simulink model "Comparacao_tomada_de_corrente_mq"  (R2024a)
settings: Solver=FixedStepAuto  StartTime=0.0  StopTime=1  FixedStep=T  RelTol=1e-3
undefined symbols (not defined in the file): J, Kf, La, T, Te, Tm, Vn
settings Model: Creator=lpds  LastModifiedBy=lpds

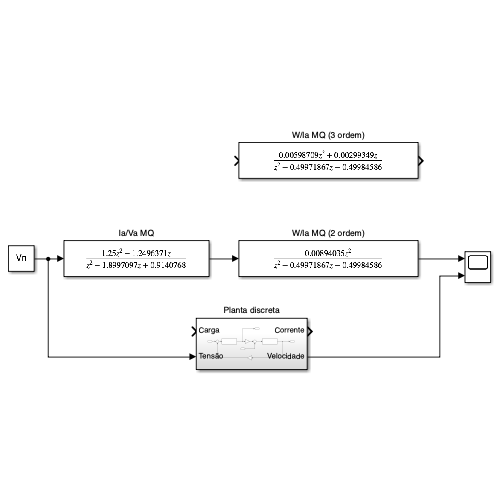
[thumbnail: Simulink's stored preview of the top-level diagram]
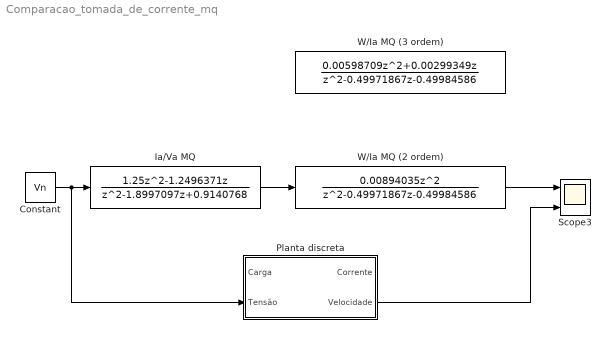
== system Comparacao_tomada_de_corrente_mq ==
  Constant : Constant  Value=Vn
  Ia/Va MQ : DiscreteTransferFcn  Numerator=[1.25, -1.2496371, 0]  Denominator=[1, -1.8997097, 0.9140768]
  Planta discreta : Subsystem
  Scope3 : Scope  NumInputPorts=2
  W/Ia MQ (2 ordem) : DiscreteTransferFcn  Numerator=[ 0.00894035, 0, 0]  Denominator=[1, -0.49971867, -0.49984586]
  W/Ia MQ (3 ordem) : DiscreteTransferFcn  Numerator=[ 0.00598709, 0.00299349, 0]  Denominator=[1, -0.49971867, -0.49984586]
  wires:
  Ia/Va MQ/1 -> W/Ia MQ (2 ordem)/1
  Planta discreta/2(Velocidade) -> Scope3/2
  Constant/1 -> Planta discreta/2(Tensão), Ia/Va MQ/1
  W/Ia MQ (2 ordem)/1 -> Scope3/1

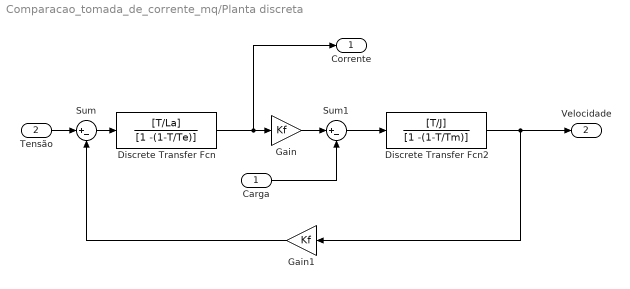
== system Comparacao_tomada_de_corrente_mq/Planta discreta ==
  Carga : Inport
  Tensão : Inport  Port=2
  Discrete Transfer Fcn : DiscreteTransferFcn  Numerator=[T/La]  Denominator=[1 -(1-T/Te)]
  Discrete Transfer Fcn2 : DiscreteTransferFcn  Numerator=[T/J]  Denominator=[1 -(1-T/Tm)]
  Gain : Gain  Gain=Kf
  Gain1 : Gain  Gain=Kf
  Sum : Sum  Inputs=|+-
  Sum1 : Sum  Inputs=|+-
  Corrente : Outport
  Velocidade : Outport  Port=2
  wires:
  Gain/1 -> Sum1/1
  Gain1/1 -> Sum/2
  Sum/1 -> Discrete Transfer Fcn/1
  Carga/1 -> Sum1/2
  Discrete Transfer Fcn2/1 -> Velocidade/1, Gain1/1
  Sum1/1 -> Discrete Transfer Fcn2/1
  Tensão/1 -> Sum/1
  Discrete Transfer Fcn/1 -> Corrente/1, Gain/1
